simulink model "simu"  (R2016a)
settings: Solver=VariableStepAuto  StartTime=0.0  StopTime=100.0  RelTol=1e-3
libraries: simulink x9
settings Model: Creator=kian  LastModifiedBy=kian

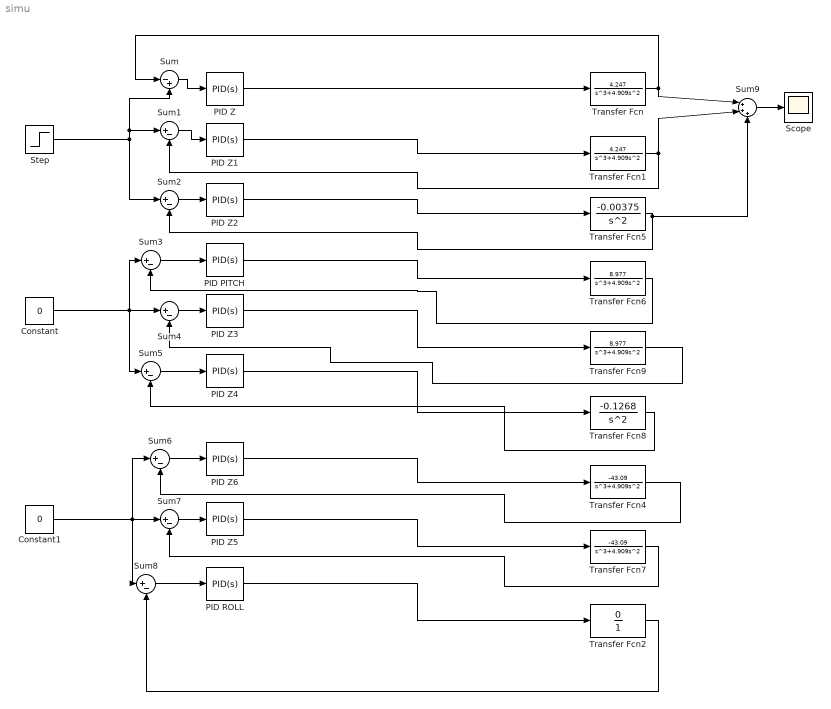
== system simu ==
  Constant : Constant  Value=0
  Constant1 : Constant  Value=0
  PID PITCH : simulink/Continuous/PID Controller  Controller=PID  TimeDomain=Continuous-time  SampleTime=-1  IntegratorMethod=Forward Euler  FilterMethod=Forward Euler  Form=Parallel  UseFilter=on  ControllerParametersSource=internal  P=1  I=1  D=0  N=100  InitialConditionSource=internal  InitialConditionForIntegrator=0  InitialConditionForFilter=0  ExternalReset=none  LimitOutput=off  UpperSaturationLimit=inf  LowerSaturationLimit=-inf  LinearizeAsGain=on  AntiWindupMode=none  Kb=1  TrackingMode=off  Kt=1  PParamMin=[]  PParamMax=[]  IParamMin=[]  IParamMax=[]  DParamMin=[]  DParamMax=[]  NParamMin=[]  NParamMax=[]  KbParamMin=[]  KbParamMax=[]  KtParamMin=[]  KtParamMax=[]  POutMin=[]  POutMax=[]  IOutMin=[]  IOutMax=[]  DOutMin=[]  DOutMax=[]  NOutMin=[]  NOutMax=[]  KbOutMin=[]  KbOutMax=[]  KtOutMin=[]  KtOutMax=[]  IntegratorOutMin=[]  IntegratorOutMax=[]  FilterOutMin=[]  FilterOutMax=[]  SumOutMin=[]  SumOutMax=[]  SumI1OutMin=[]  SumI1OutMax=[]  SumI2OutMin=[]  SumI2OutMax=[]  SumI3OutMin=[]  SumI3OutMax=[]  SumDOutMin=[]  SumDOutMax=[]  SaturationOutMin=[]  SaturationOutMax=[]  IntegratorContinuousStateAttributes=''  IntegratorStateMustResolveToSignalObject=off  IntegratorRTWStateStorageClass=Auto  FilterContinuousStateAttributes=''  FilterStateMustResolveToSignalObject=off  FilterRTWStateStorageClass=Auto  DifferentiatorICPrevScaledInput=0  DifferentiatorOutMin=[]  DifferentiatorOutMax=[]
  PID ROLL : simulink/Continuous/PID Controller  Controller=PID  TimeDomain=Continuous-time  SampleTime=-1  IntegratorMethod=Forward Euler  FilterMethod=Forward Euler  Form=Parallel  UseFilter=on  ControllerParametersSource=internal  P=1  I=1  D=0  N=100  InitialConditionSource=internal  InitialConditionForIntegrator=0  InitialConditionForFilter=0  ExternalReset=none  LimitOutput=off  UpperSaturationLimit=inf  LowerSaturationLimit=-inf  LinearizeAsGain=on  AntiWindupMode=none  Kb=1  TrackingMode=off  Kt=1  PParamMin=[]  PParamMax=[]  IParamMin=[]  IParamMax=[]  DParamMin=[]  DParamMax=[]  NParamMin=[]  NParamMax=[]  KbParamMin=[]  KbParamMax=[]  KtParamMin=[]  KtParamMax=[]  POutMin=[]  POutMax=[]  IOutMin=[]  IOutMax=[]  DOutMin=[]  DOutMax=[]  NOutMin=[]  NOutMax=[]  KbOutMin=[]  KbOutMax=[]  KtOutMin=[]  KtOutMax=[]  IntegratorOutMin=[]  IntegratorOutMax=[]  FilterOutMin=[]  FilterOutMax=[]  SumOutMin=[]  SumOutMax=[]  SumI1OutMin=[]  SumI1OutMax=[]  SumI2OutMin=[]  SumI2OutMax=[]  SumI3OutMin=[]  SumI3OutMax=[]  SumDOutMin=[]  SumDOutMax=[]  SaturationOutMin=[]  SaturationOutMax=[]  IntegratorContinuousStateAttributes=''  IntegratorStateMustResolveToSignalObject=off  IntegratorRTWStateStorageClass=Auto  FilterContinuousStateAttributes=''  FilterStateMustResolveToSignalObject=off  FilterRTWStateStorageClass=Auto  DifferentiatorICPrevScaledInput=0  DifferentiatorOutMin=[]  DifferentiatorOutMax=[]
  PID Z{,1..6} (7 alike) : simulink/Continuous/PID Controller  Controller=PID  TimeDomain=Continuous-time  SampleTime=-1  IntegratorMethod=Forward Euler  FilterMethod=Forward Euler  Form=Parallel  UseFilter=on  ControllerParametersSource=internal  P=1  I=1  D=0  N=100  InitialConditionSource=internal  InitialConditionForIntegrator=0  InitialConditionForFilter=0  ExternalReset=none  LimitOutput=off  UpperSaturationLimit=inf  LowerSaturationLimit=-inf  LinearizeAsGain=on  AntiWindupMode=none  Kb=1  TrackingMode=off  Kt=1  PParamMin=[]  PParamMax=[]  IParamMin=[]  IParamMax=[]  DParamMin=[]  DParamMax=[]  NParamMin=[]  NParamMax=[]  KbParamMin=[]  KbParamMax=[]  KtParamMin=[]  KtParamMax=[]  POutMin=[]  POutMax=[]  IOutMin=[]  IOutMax=[]  DOutMin=[]  DOutMax=[]  NOutMin=[]  NOutMax=[]  KbOutMin=[]  KbOutMax=[]  KtOutMin=[]  KtOutMax=[]  IntegratorOutMin=[]  IntegratorOutMax=[]  FilterOutMin=[]  FilterOutMax=[]  SumOutMin=[]  SumOutMax=[]  SumI1OutMin=[]  SumI1OutMax=[]  SumI2OutMin=[]  SumI2OutMax=[]  SumI3OutMin=[]  SumI3OutMax=[]  SumDOutMin=[]  SumDOutMax=[]  SaturationOutMin=[]  SaturationOutMax=[]  IntegratorContinuousStateAttributes=''  IntegratorStateMustResolveToSignalObject=off  IntegratorRTWStateStorageClass=Auto  FilterContinuousStateAttributes=''  FilterStateMustResolveToSignalObject=off  FilterRTWStateStorageClass=Auto  DifferentiatorICPrevScaledInput=0  DifferentiatorOutMin=[]  DifferentiatorOutMax=[]
  Scope : Scope
  Step : Step  SampleTime=0
  Sum : Sum  Inputs=|-+
  Sum{1..8} (8 alike) : Sum  Inputs=|+-
  Sum9 : Sum  Inputs=|+++
  Transfer Fcn : TransferFcn  Numerator=[4.247]  Denominator=[1 4.909 0 0]
  Transfer Fcn1 : TransferFcn  Numerator=[4.247]  Denominator=[1 4.909 0 0]
  Transfer Fcn2 : TransferFcn  Numerator=[0]  Denominator=[1]
  Transfer Fcn4 : TransferFcn  Numerator=[-43.09]  Denominator=[1 4.909 0 0]
  Transfer Fcn5 : TransferFcn  Numerator=[-0.00375]  Denominator=[1 0 0]
  Transfer Fcn6 : TransferFcn  Numerator=[8.977]  Denominator=[1 4.909 0 0]
  Transfer Fcn7 : TransferFcn  Numerator=[-43.09]  Denominator=[1 4.909 0 0]
  Transfer Fcn8 : TransferFcn  Numerator=[-0.1268]  Denominator=[1 0 0]
  Transfer Fcn9 : TransferFcn  Numerator=[8.977]  Denominator=[1 4.909 0 0]
  wires:
  Constant1/1 -> Sum8/1, Sum7/1, Sum6/1
  Step/1 -> Sum2/1, Sum1/1, Sum/2
  PID Z/1 -> Transfer Fcn/1
  PID Z1/1 -> Transfer Fcn1/1
  PID Z2/1 -> Transfer Fcn5/1
  PID PITCH/1 -> Transfer Fcn6/1
  PID Z3/1 -> Transfer Fcn9/1
  PID Z4/1 -> Transfer Fcn8/1
  PID Z6/1 -> Transfer Fcn4/1
  PID Z5/1 -> Transfer Fcn7/1
  PID ROLL/1 -> Transfer Fcn2/1
  Transfer Fcn/1 -> Sum9/1, Sum/1
  Transfer Fcn1/1 -> Sum1/2, Sum9/2
  Sum/1 -> PID Z/1
  Sum1/1 -> PID Z1/1
  Transfer Fcn5/1 -> Sum9/3, Sum2/2
  Sum2/1 -> PID Z2/1
  Sum3/1 -> PID PITCH/1
  Transfer Fcn6/1 -> Sum3/2
  Sum4/1 -> PID Z3/1
  Transfer Fcn9/1 -> Sum4/2
  Constant/1 -> Sum5/1, Sum4/1, Sum3/1
  Sum5/1 -> PID Z4/1
  Transfer Fcn8/1 -> Sum5/2
  Sum6/1 -> PID Z6/1
  Transfer Fcn4/1 -> Sum6/2
  Sum7/1 -> PID Z5/1
  Transfer Fcn7/1 -> Sum7/2
  Sum8/1 -> PID ROLL/1
  Transfer Fcn2/1 -> Sum8/2
  Sum9/1 -> Scope/1
